simulink model "Prob7"  (R2020b)
settings: Solver=VariableStepAuto  StartTime=0.0  StopTime=10.0  RelTol=1e-3
settings Model: Creator=stkaravind  LastModifiedBy=stkaravind

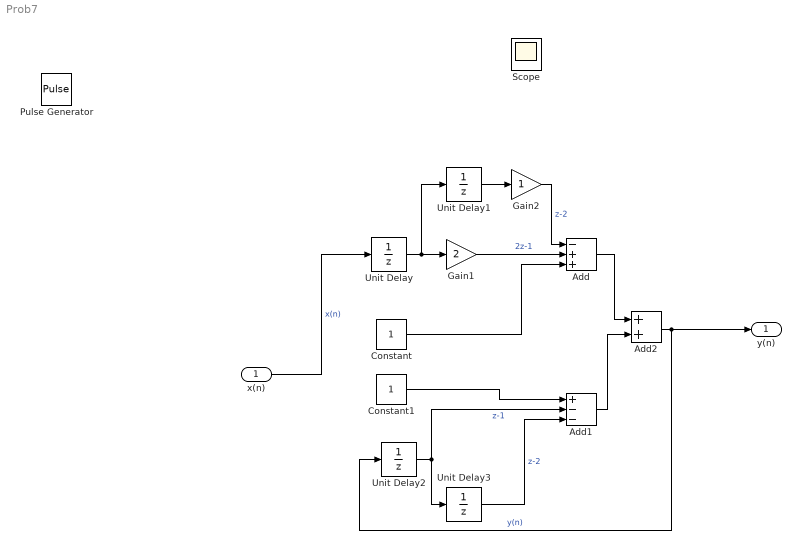
== system Prob7 ==
  x(n) : Inport  OutDataTypeStr=double  PortDimensions=1  SampleTime=[0,1]
  Add : Sum  Inputs=-++
  Add1 : Sum  Inputs=+--
  Add2 : Sum
  Constant : Constant
  Constant1 : Constant
  Gain1 : Gain  Gain=2
  Gain2 : Gain
  Pulse Generator : DiscretePulseGenerator  PulseType=Time based  Period=10  PulseWidth=5
  Scope : Scope
  Unit Delay{,1..3} (4 alike) : UnitDelay  SampleTime=-1  HasFrameUpgradeWarning=on
  y(n) : Outport  OutDataTypeStr=double  PortDimensions=1  SampleTime=[2,0]
  wires:
  Add2/1 -> Unit Delay2/1, y(n)/1  "y(n)"
  Unit Delay1/1 -> Gain2/1
  Constant1/1 -> Add1/1
  x(n)/1 -> Unit Delay/1  "x(n)"
  Unit Delay3/1 -> Add1/3  "z-2"
  Add/1 -> Add2/1
  Gain1/1 -> Add/2  "2z-1"
  Gain2/1 -> Add/1  "z-2"
  Unit Delay2/1 -> Add1/2, Unit Delay3/1  "z-1"
  Unit Delay/1 -> Gain1/1, Unit Delay1/1
  Constant/1 -> Add/3
  Add1/1 -> Add2/2
